simulink model "lqr_2dof_nonlinear_c_speed"  (R2017a)
settings: Solver=ode45  StartTime=0.0  StopTime=5  RelTol=1e-3
undefined symbols (not defined in the file): f, g, GoalPos, K, k_p, l, m_p
settings Model: Creator=sansh  LastModifiedBy=rj2318

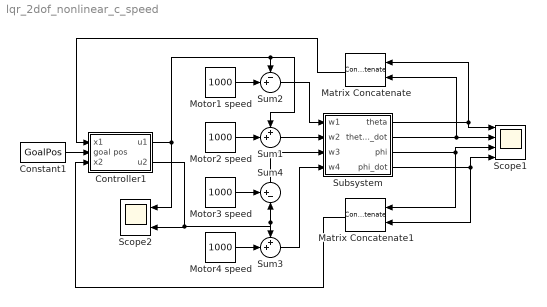
== system lqr_2dof_nonlinear_c_speed ==
  Constant1 : Constant  Value=GoalPos
  Controller1 : Subsystem
  Matrix Concatenate : Concatenate  Mode=Multidimensional array  ConcatenateDimension=2
  Matrix Concatenate1 : Concatenate  Mode=Multidimensional array  ConcatenateDimension=2
  Motor1 speed : Constant  Value=1000
  Motor2 speed : Constant  Value=1000
  Motor3 speed : Constant  Value=1000
  Motor4 speed : Constant  Value=1000
  Scope1 : Scope  NumInputPorts=4
  Scope2 : Scope  NumInputPorts=2
  Subsystem : Subsystem
  Sum1 : Sum  Inputs=++|
  Sum2 : Sum  Inputs=-+|
  Sum3 : Sum  Inputs=++|
  Sum4 : Sum  Inputs=+-|
  wires:
  Matrix Concatenate/1 -> Controller1/1(x1)
  Constant1/1 -> Controller1/2(goal pos)
  Subsystem/3(phi) -> Scope1/3, Matrix Concatenate1/1
  Subsystem/2(theta_dot) -> Matrix Concatenate/2, Scope1/2
  Matrix Concatenate1/1 -> Controller1/3(x2)
  Subsystem/4(phi_dot) -> Matrix Concatenate1/2, Scope1/4
  Subsystem/1(theta) -> Matrix Concatenate/1, Scope1/1
  Sum3/1 -> Subsystem/4(w4)
  Controller1/2(u2) -> Scope2/2, Sum4/2, Sum3/1
  Sum2/1 -> Subsystem/1(w1)
  Sum1/1 -> Subsystem/2(w2)
  Sum4/1 -> Subsystem/3(w3)
  Motor1 speed/1 -> Sum2/2
  Controller1/1(u1) -> Scope2/1, Sum1/1, Sum2/1
  Motor4 speed/1 -> Sum3/2
  Motor2 speed/1 -> Sum1/2
  Motor3 speed/1 -> Sum4/1

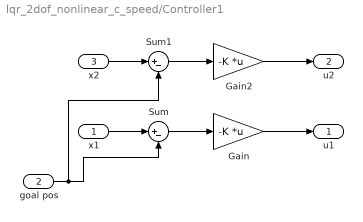
== system lqr_2dof_nonlinear_c_speed/Controller1 ==
  x1 : Inport
  goal pos : Inport  Port=2
  x2 : Inport  Port=3
  Gain : Gain  Gain=-K  Multiplication=Matrix(K*u)
  Gain2 : Gain  Gain=-K  Multiplication=Matrix(K*u)
  Sum : Sum  Inputs=|+-
  Sum1 : Sum  Inputs=|+-
  u1 : Outport
  u2 : Outport  Port=2
  wires:
  x1/1 -> Sum/1
  Gain/1 -> u1/1
  Sum/1 -> Gain/1
  Gain2/1 -> u2/1
  Sum1/1 -> Gain2/1
  goal pos/1 -> Sum1/2, Sum/2
  x2/1 -> Sum1/1

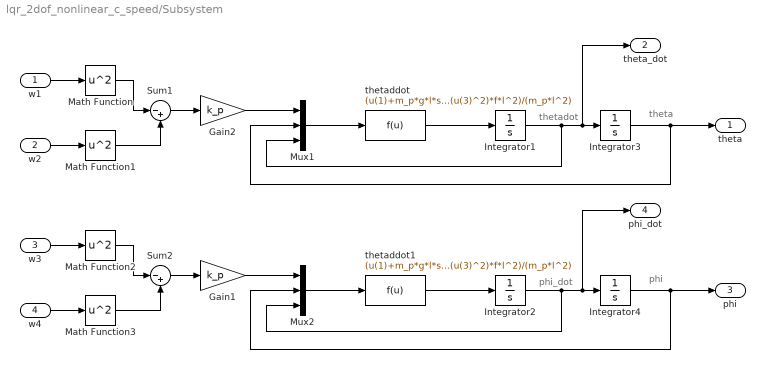
== system lqr_2dof_nonlinear_c_speed/Subsystem ==
  note: theta
  note: thetadot
  note: phi
  note: phi_dot
  w1 : Inport
  w2 : Inport  Port=2
  w3 : Inport  Port=3
  w4 : Inport  Port=4
  Gain1 : Gain  Gain=k_p
  Gain2 : Gain  Gain=k_p
  Integrator1 : Integrator  ContinuousStateAttributes='thetadot'
  Integrator2 : Integrator  ContinuousStateAttributes='thetadot'
  Integrator3 : Integrator  InitialCondition=0.1  ContinuousStateAttributes='theta'
  Integrator4 : Integrator  InitialCondition=0.1  ContinuousStateAttributes='theta'
  Math Function{,1..3} (4 alike) : Math  Operator=square  SaturateOnIntegerOverflow=on
  Mux1 : Mux  Inputs=3
  Mux2 : Mux  Inputs=3
  Sum1 : Sum  Inputs=|-+
  Sum2 : Sum  Inputs=|-+
  thetaddot : Fcn  Expr=(u(1)+m_p*g*l*sin(u(2))-(u(3)^2)*f*l^2)/(m_p*l^2)
  thetaddot1 : Fcn  Expr=(u(1)+m_p*g*l*sin(u(2))-(u(3)^2)*f*l^2)/(m_p*l^2)
  theta : Outport
  theta_dot : Outport  Port=2
  phi : Outport  Port=3
  phi_dot : Outport  Port=4
  wires:
  Mux1/1 -> thetaddot/1
  thetaddot/1 -> Integrator1/1
  Integrator1/1 -> Mux1/3, theta_dot/1, Integrator3/1
  Integrator3/1 -> Mux1/2, theta/1
  Integrator4/1 -> Mux2/2, phi/1
  thetaddot1/1 -> Integrator2/1
  Mux2/1 -> thetaddot1/1
  Integrator2/1 -> Mux2/3, phi_dot/1, Integrator4/1
  w2/1 -> Math Function1/1
  Gain2/1 -> Mux1/1
  Sum1/1 -> Gain2/1
  Math Function/1 -> Sum1/1
  Math Function1/1 -> Sum1/2
  w1/1 -> Math Function/1
  w4/1 -> Math Function3/1
  Gain1/1 -> Mux2/1
  Sum2/1 -> Gain1/1
  Math Function2/1 -> Sum2/1
  Math Function3/1 -> Sum2/2
  w3/1 -> Math Function2/1
